simulink model "Simplified_L1F_SPp"  (R2016a)
settings: Solver=VariableStepDiscrete  StartTime=0.0  StopTime=2e-3  MaxStep=8.145975887911372E-11  RelTol=1e-3
InitFcn:
  | SampleFreq = 122.76e6;
  | Sample_Time = 1/SampleFreq;
  | Integration_time = 1e-3;
undefined symbols (not defined in the file): c1, c2, magnitude
libraries: commfilt2 x6, dspsigops x5, commseqgen3 x4
settings Model: Creator=User  LastModifiedBy=User
settings DataIOCC: InspectSignalLogs=on

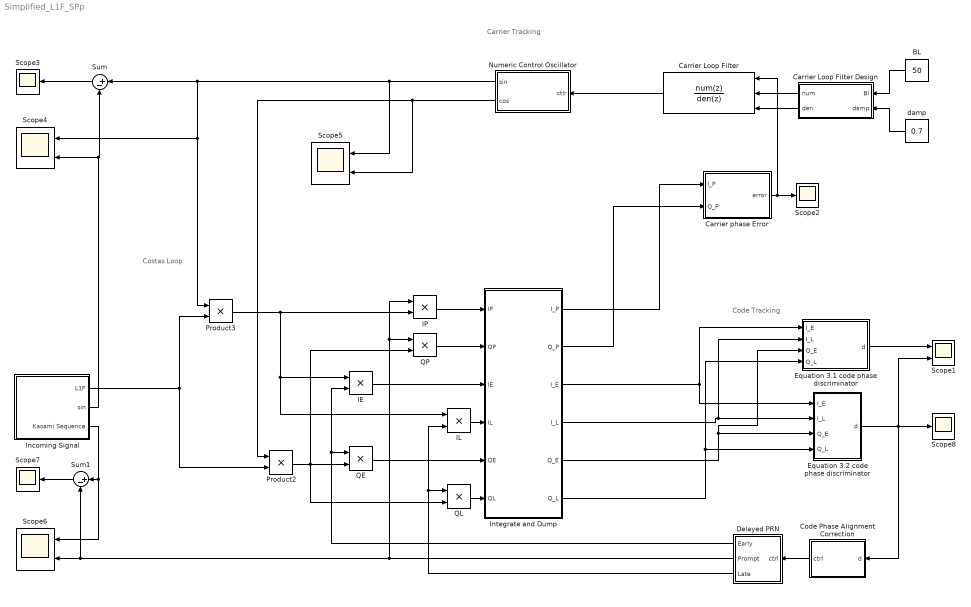
== system Simplified_L1F_SPp ==
  note: Costas Loop
  note: Carrier Tracking
  note: Code Tracking
  BL : Constant  Value=50
  Carrier Loop Filter Design : MATLAB Function  TreatAsAtomicUnit=on
  Carrier Loop Filter : DiscreteFilter  NumeratorSource=Input port  Numerator=c1+c2  DenominatorSource=Input port  Denominator=[1 -1 1]  FilterStructure=Direct form I  SampleTime=Integration_time  a0EqualsOne=on  NumProductDataTypeStr=fixdt(1,16,0)  DenProductDataTypeStr=fixdt(1,16,0)  NumAccumDataTypeStr=fixdt(1,16,0)  DenAccumDataTypeStr=fixdt(1,16,0)  OutDataTypeStr=fixdt(1,16,0)  SaturateOnIntegerOverflow=on
      settings: InputPortMap=u0,p1,p3  LockScale=on
  Carrier phase Error : MATLAB Function  TreatAsAtomicUnit=on
  Code Phase Alignment Correction : MATLAB Function  TreatAsAtomicUnit=on
  Delayed PRN : Subsystem
  Equation 3.1 code phase discriminator : MATLAB Function  TreatAsAtomicUnit=on
  Equation 3.2 code phase discriminator : Subsystem
  IE : Product
  IL : Product
  IP : Product
  Incoming Signal : Subsystem
  Integrate and Dump : Subsystem
  Numeric Control Oscillator : Subsystem
  Product2 : Product
  Product3 : Product
  QE : Product
  QL : Product
  QP : Product
  Scope{1,4..6} (4 alike) : Scope  NumInputPorts=2
  Scope{2..3,7..8} (4 alike) : Scope
  Sum : Sum  Inputs=|+-
  Sum1 : Sum  Inputs=|+-
  damp : Constant  Value=0.7
  wires:
  Code Phase Alignment Correction/1(ctrl) -> Delayed PRN/1(ctrl)
  Equation 3.2 code phase discriminator/1(d) -> Scope8/1, Scope1/2, Code Phase Alignment Correction/1(d)
  Equation 3.1 code phase discriminator/1(d) -> Scope1/1
  Carrier phase Error/1(error) -> Carrier Loop Filter/1, Scope2/1
  QL/1 -> Integrate and Dump/6(QL)
  IL/1 -> Integrate and Dump/4(IL)
  IP/1 -> Integrate and Dump/1(IP)
  QP/1 -> Integrate and Dump/2(QP)
  QE/1 -> Integrate and Dump/5(QE)
  IE/1 -> Integrate and Dump/3(IE)
  Product3/1 -> IL/1, IE/1, IP/2
  Product2/1 -> QL/2, QP/2, QE/2
  Delayed PRN/3(Late) -> IL/2, QL/1
  Delayed PRN/2(Prompt) -> Scope6/2, Sum1/2, IP/1, QP/1
  Delayed PRN/1(Early) -> IE/2, QE/1
  Incoming Signal/1(L1F) -> Product2/2, Product3/2
  Numeric Control Oscillator/1(sin) -> Scope5/1, Sum/1, Product3/1, Scope4/1
  Numeric Control Oscillator/2(cos) -> Scope5/2, Product2/1
  Incoming Signal/2(sin) -> Scope4/2, Sum/2
  Sum/1 -> Scope3/1
  Incoming Signal/3("Kasami Sequence ") -> Sum1/1, Scope6/1
  Sum1/1 -> Scope7/1
  BL/1 -> Carrier Loop Filter Design/1(Bl)
  damp/1 -> Carrier Loop Filter Design/2(damp)
  Carrier Loop Filter Design/1(num) -> Carrier Loop Filter/2
  Carrier Loop Filter Design/2(den) -> Carrier Loop Filter/3
  Integrate and Dump/1(I_P) -> Carrier phase Error/1(I_P)
  Integrate and Dump/2(Q_P) -> Carrier phase Error/2(Q_P)
  Integrate and Dump/3(I_E) -> Equation 3.2 code phase discriminator/1(I_E), Equation 3.1 code phase discriminator/1(I_E)
  Integrate and Dump/4(I_L) -> Equation 3.1 code phase discriminator/2(I_L), Equation 3.2 code phase discriminator/2(I_L)
  Integrate and Dump/5(Q_E) -> Equation 3.2 code phase discriminator/3(Q_E), Equation 3.1 code phase discriminator/3(Q_E)
  Integrate and Dump/6(Q_L) -> Equation 3.2 code phase discriminator/4(Q_L), Equation 3.1 code phase discriminator/4(Q_L)
  Carrier Loop Filter/1 -> Numeric Control Oscillator/1(ctlr)

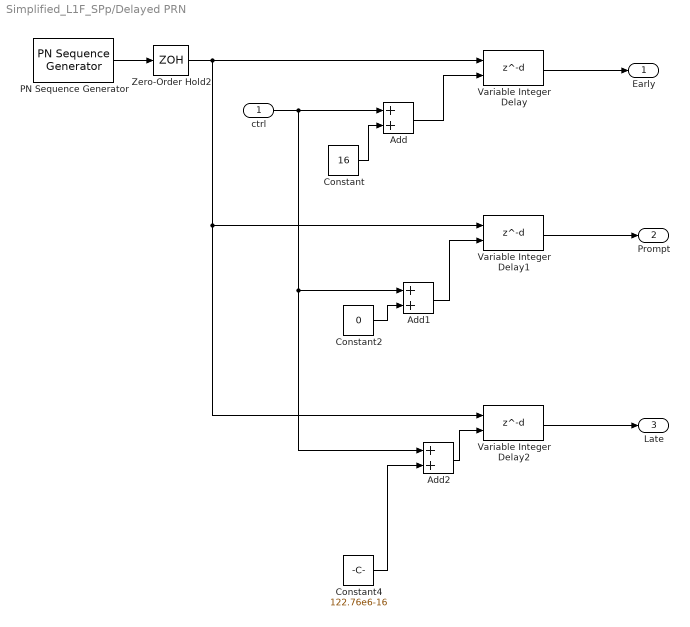
== system Simplified_L1F_SPp/Delayed PRN ==
  ctrl : Inport
  Add : Sum
  Add1 : Sum
  Add2 : Sum
  Constant : Constant  Value=16  SampleTime=Sample_Time
  Constant2 : Constant  Value=0  SampleTime=Sample_Time
  Constant4 : Constant  Value=122.76e6-16  SampleTime=Sample_Time
  PN Sequence Generator : commseqgen3/PN Sequence Generator  poly='z^9 + z^4 + 1'  ini_sta=ones(1,9)  outBitMaskSource=Dialog parameter  shift=7  outVarSiz=off  maxOutSizeMode=Dialog parameter  maxOutSize=[10 1]  Ts=1e-3/511  sampPerFrame=1  reset=off  bitPackedOutputs=off  outDataType=double  numPackedBits=8  bitPackDataSigned=off  bitPackedOutDType=double
  Variable Integer Delay : Delay  DelayLengthSource=Input port
      settings: InputPortMap=u0,p1
  Variable Integer Delay1 : Delay  DelayLengthSource=Input port
      settings: InputPortMap=u0,p1
  Variable Integer Delay2 : Delay  DelayLengthSource=Input port
      settings: InputPortMap=u0,p1
  Zero-Order Hold2 : ZeroOrderHold  SampleTime=Sample_Time
  Early : Outport
  Prompt : Outport  Port=2
  Late : Outport  Port=3
  wires:
  Constant/1 -> Add/2
  Add1/1 -> Variable Integer Delay1/2
  Add/1 -> Variable Integer Delay/2
  ctrl/1 -> Add2/1, Add1/1, Add/1
  Constant2/1 -> Add1/2
  Constant4/1 -> Add2/2
  Add2/1 -> Variable Integer Delay2/2
  Variable Integer Delay/1 -> Early/1
  Variable Integer Delay1/1 -> Prompt/1
  Variable Integer Delay2/1 -> Late/1
  PN Sequence Generator/1 -> Zero-Order Hold2/1
  Zero-Order Hold2/1 -> Variable Integer Delay1/1, Variable Integer Delay2/1, Variable Integer Delay/1

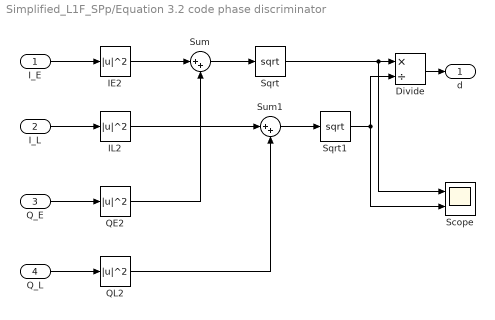
== system Simplified_L1F_SPp/Equation 3.2 code phase discriminator ==
  I_E : Inport
  I_L : Inport  Port=2
  Q_E : Inport  Port=3
  Q_L : Inport  Port=4
  Divide : Product  Inputs=*/
  IE2 : Math  Operator=magnitude^2  SaturateOnIntegerOverflow=on
  IL2 : Math  Operator=magnitude^2  SaturateOnIntegerOverflow=on
  QE2 : Math  Operator=magnitude^2  SaturateOnIntegerOverflow=on
  QL2 : Math  Operator=magnitude^2  SaturateOnIntegerOverflow=on
  Scope : Scope  NumInputPorts=2
  Sqrt : Sqrt  SaturateOnIntegerOverflow=on
  Sqrt1 : Sqrt  SaturateOnIntegerOverflow=on
  Sum : Sum  Inputs=|++
  Sum1 : Sum  Inputs=|++
  d : Outport
  wires:
  IE2/1 -> Sum/1
  QE2/1 -> Sum/2
  Sum/1 -> Sqrt/1
  IL2/1 -> Sum1/1
  Sqrt/1 -> Scope/1, Divide/1
  QL2/1 -> Sum1/2
  Sqrt1/1 -> Scope/2, Divide/2
  Sum1/1 -> Sqrt1/1
  I_L/1 -> IL2/1
  Q_L/1 -> QL2/1
  Q_E/1 -> QE2/1
  I_E/1 -> IE2/1
  Divide/1 -> d/1

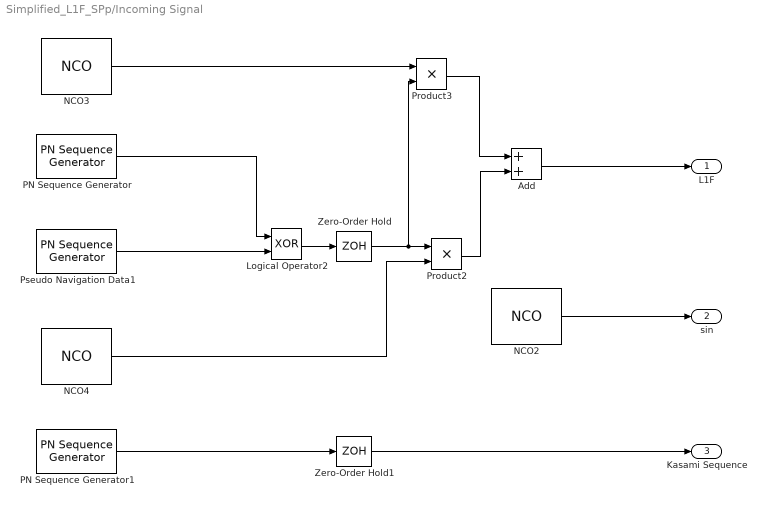
== system Simplified_L1F_SPp/Incoming Signal ==
  Add : Sum
  Logical Operator2 : Logic  Operator=XOR  AllPortsSameDT=off  OutDataTypeStr=boolean
  NCO2 : dspsigops/NCO  AccIncSrc=Specify via dialog  AccInc=100  PhaseOffsetSrc=Specify via dialog  PhaseOffset=0  AccumWL=16  HasDither=off  DitherWL=4  PNgeneratorLength=19  HasPhaseQuantizer=on  TableDepth=14  HasOutputPhaseError=off  Formula=Sine  DataType=Binary point scaling  OutputWL=16  OutputFL=14  CompMethod=Table lookup (no interpolation)  SampleTime=Sample_Time  SamplesPerFrame=1  OutputFrames=off
  NCO3 : dspsigops/NCO  AccIncSrc=Specify via dialog  AccInc=100  PhaseOffsetSrc=Specify via dialog  PhaseOffset=0  AccumWL=16  HasDither=off  DitherWL=4  PNgeneratorLength=19  HasPhaseQuantizer=on  TableDepth=14  HasOutputPhaseError=off  Formula=Sine  DataType=Binary point scaling  OutputWL=16  OutputFL=14  CompMethod=Table lookup (no interpolation)  SampleTime=Sample_Time  SamplesPerFrame=1  OutputFrames=off
  NCO4 : dspsigops/NCO  AccIncSrc=Specify via dialog  AccInc=100  PhaseOffsetSrc=Specify via dialog  PhaseOffset=0  AccumWL=16  HasDither=off  DitherWL=4  PNgeneratorLength=19  HasPhaseQuantizer=on  TableDepth=14  HasOutputPhaseError=off  Formula=Cosine  DataType=Binary point scaling  OutputWL=16  OutputFL=14  CompMethod=Table lookup (no interpolation)  SampleTime=Sample_Time  SamplesPerFrame=1  OutputFrames=off
  PN Sequence Generator : commseqgen3/PN Sequence Generator  poly='z^9 + z^4 + 1'  ini_sta=ones(1,9)  outBitMaskSource=Dialog parameter  shift=7  outVarSiz=off  maxOutSizeMode=Dialog parameter  maxOutSize=[10 1]  Ts=1e-3/511  sampPerFrame=1  reset=off  bitPackedOutputs=off  outDataType=double  numPackedBits=8  bitPackDataSigned=off  bitPackedOutDType=double
  PN Sequence Generator1 : commseqgen3/PN Sequence Generator  poly='z^9 + z^4 + 1'  ini_sta=ones(1,9)  outBitMaskSource=Dialog parameter  shift=7  outVarSiz=off  maxOutSizeMode=Dialog parameter  maxOutSize=[10 1]  Ts=1e-3/511  sampPerFrame=1  reset=off  bitPackedOutputs=off  outDataType=double  numPackedBits=8  bitPackDataSigned=off  bitPackedOutDType=double
  Product2 : Product
  Product3 : Product
  Pseudo Navigation Data1 : commseqgen3/PN Sequence Generator  poly='z^14 + z^13 + z^8 + z^4 + 1'  ini_sta=[0 0 1 1 0 1 0 0 1 1 1 0 0 0]  outBitMaskSource=Dialog parameter  shift=14  outVarSiz=off  maxOutSizeMode=Dialog parameter  maxOutSize=[10 1]  Ts=1/50  sampPerFrame=1  reset=off  bitPackedOutputs=off  outDataType=double  numPackedBits=8  bitPackDataSigned=off  bitPackedOutDType=double
  Zero-Order Hold : ZeroOrderHold  SampleTime=Sample_Time
  Zero-Order Hold1 : ZeroOrderHold  SampleTime=Sample_Time
  L1F : Outport
  sin : Outport  Port=2
  "Kasami Sequence " : Outport  Port=3
  wires:
  NCO4/1 -> Product2/2
  PN Sequence Generator/1 -> Logical Operator2/1
  NCO3/1 -> Product3/1
  Logical Operator2/1 -> Zero-Order Hold/1
  Add/1 -> L1F/1
  PN Sequence Generator1/1 -> Zero-Order Hold1/1
  NCO2/1 -> sin/1
  Product3/1 -> Add/1
  Product2/1 -> Add/2
  Zero-Order Hold/1 -> Product3/2, Product2/1
  Zero-Order Hold1/1 -> "Kasami Sequence "/1
  Pseudo Navigation Data1/1 -> Logical Operator2/2

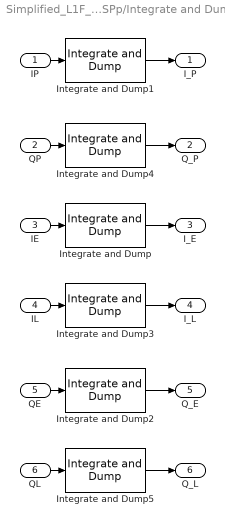
== system Simplified_L1F_SPp/Integrate and Dump ==
  IP : Inport
  QP : Inport  Port=2
  IE : Inport  Port=3
  IL : Inport  Port=4
  QE : Inport  Port=5
  QL : Inport  Port=6
  Integrate and Dump{,1..5} (6 alike) : commfilt2/Integrate and Dump  obssamples=SampleFreq*Integration_time  offsetsamples=0  nodump=off  roundingMode=Floor  overflowMode=off  outputDataTypeStr=Inherit: Same as accumulator  outputLastDataTypeStr=Inherit: Same as accumulator
  I_P : Outport
  Q_P : Outport  Port=2
  I_E : Outport  Port=3
  I_L : Outport  Port=4
  Q_E : Outport  Port=5
  Q_L : Outport  Port=6
  wires:
  IP/1 -> Integrate and Dump1/1
  QP/1 -> Integrate and Dump4/1
  IE/1 -> Integrate and Dump/1
  IL/1 -> Integrate and Dump3/1
  QE/1 -> Integrate and Dump2/1
  QL/1 -> Integrate and Dump5/1
  Integrate and Dump1/1 -> I_P/1
  Integrate and Dump4/1 -> Q_P/1
  Integrate and Dump5/1 -> Q_L/1
  Integrate and Dump2/1 -> Q_E/1
  Integrate and Dump3/1 -> I_L/1
  Integrate and Dump/1 -> I_E/1

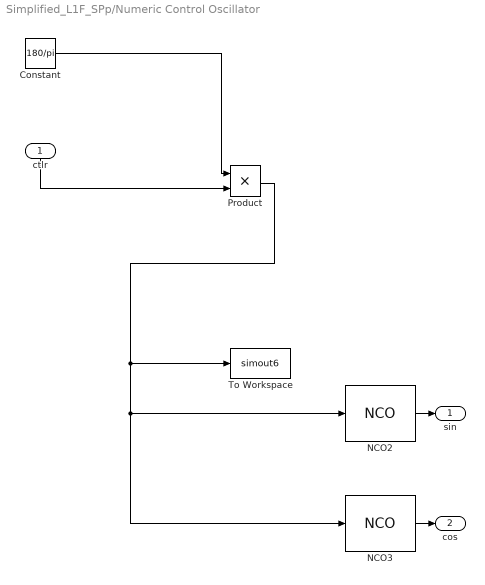
== system Simplified_L1F_SPp/Numeric Control Oscillator ==
  ctlr : Inport
  Constant : Constant  Value=180/pi  OutDataTypeStr=fixdt(1,16,0)  SampleTime=Integration_time
  NCO2 : dspsigops/NCO  AccIncSrc=Input port  AccInc=100  PhaseOffsetSrc=Specify via dialog  PhaseOffset=0  AccumWL=16  HasDither=off  DitherWL=4  PNgeneratorLength=19  HasPhaseQuantizer=on  TableDepth=14  HasOutputPhaseError=off  Formula=Sine  DataType=Binary point scaling  OutputWL=16  OutputFL=14  CompMethod=Table lookup (no interpolation)  SampleTime=1  SamplesPerFrame=1  OutputFrames=off
  NCO3 : dspsigops/NCO  AccIncSrc=Input port  AccInc=100  PhaseOffsetSrc=Specify via dialog  PhaseOffset=0  AccumWL=16  HasDither=off  DitherWL=4  PNgeneratorLength=19  HasPhaseQuantizer=on  TableDepth=14  HasOutputPhaseError=off  Formula=Cosine  DataType=Binary point scaling  OutputWL=16  OutputFL=14  CompMethod=Table lookup (no interpolation)  SampleTime=1  SamplesPerFrame=1  OutputFrames=off
  Product : Product
  To Workspace : ToWorkspace  VariableName=simout6  SampleTime=-1
      settings: Save2DSignal=2-D array (concatenate along first dimension)
  sin : Outport
  cos : Outport  Port=2
  wires:
  NCO3/1 -> cos/1
  NCO2/1 -> sin/1
  Product/1 -> NCO2/1, NCO3/1, To Workspace/1
  ctlr/1 -> Product/2
  Constant/1 -> Product/1

== matlab function Simplified_L1F_SPp/Equation 3.1 code phase discriminator ==
  data: I_E input; d output; I_L input; Q_E input; Q_L input
function d = fcn(I_E,I_L,Q_E,Q_L)
d = ((I_E^2+Q_E^2)-(I_L^2+Q_L^2))/((I_E^2+Q_E^2)+(I_L^2+Q_L^2));
end

== matlab function Simplified_L1F_SPp/Code Phase Alignment Correction ==
  data: d input; ctrl output
function ctrl = fcn(d)
    ctrl = 0;
    if d > 1.5
    ctrl = ctrl - 1; 
    elseif d < 0.8
    ctrl = ctrl + 1; 
    else
    ctrl = ctrl + 0; 
    end
end

== matlab function Simplified_L1F_SPp/Carrier phase Error ==
  data: I_P input; error output; Q_P input
function error = fcn(I_P,Q_P)
TbAn = [0 1 2 3 4 5 6 7 8 9 10 11 12 13 14 15 16 17 18 19 20 21 22 23 24 25 26 27 28 29 30 31 32 33 34 35 36 37 38 39 40 41 42 43 44 45 46 47 48 49 50 51 52 52 53 54 55 56 57 58 59 60 61 61 62 63 64 65 66 67 68 68 69 70 71 72 73 73 74 75 76 77 78 78 79 80 81 82 82 83 84 85 85 86 87 88 89 89 90 91 91 92 93 94 94 95 96 97 97 98 99 99 100 101 101 102 103 103 104 105 105 106 107 107 108 109 109 110 110 111 112 112 113 114 114 115 115 116 116 117 118 118 119 119 120 120 121 122 122 123 123 124 124 125 125 126 126 127 127 128];
if  (I_P < 0) 
     I_P = -I_P; 
     Q_P = -Q_P; 
end

mRe = abs(I_P); 
mIm = abs(Q_P);

if (mRe >= mIm)
   Ph = TbAn(ceil((mIm*159)/mRe));	
else 
   Ph = 256 - TbAn(ceil((mRe*159)/mIm));				
end
error = 0;
if I_P == 0 
       if Q_P > 0 
            error= 256;
       elseif Q_P < 0 
            error= -256;
       end
elseif I_P < 0 
       if Q_P >= 0
          error= 512-Ph;
       elseif Q_P > 0
       error = -512+Ph;
       end
elseif I_P > 0
       if Q_P >= 0 
          error= Ph;
       elseif Q_P<0
          error = -Ph;
       end
end
error = error*pi/180;
end

== matlab function Simplified_L1F_SPp/Carrier Loop Filter Design ==
  data: Bl input; num output; damp input; den output
function [num, den]= fcn(Bl, damp)
    wn = 8*Bl*damp/(4*damp*damp+1);
    dT = 1e-3;
    k = 400*pi;
    c1 = 1/k*8*damp*wn*dT/(4+4*damp*wn*dT+wn*wn*dT*dT);
    c2 = 1/k*4*wn*wn*dT*dT/(4+4*damp*wn*dT+wn*wn*dT*dT);
    num = [c1+c2 -c1];
    den = [1 -1];
end
